simulink model "ship_template"  (R2021b)
settings: Solver=ode23t  StartTime=0.0  StopTime=60*2  MaxStep=0.1  RelTol=1e-3  AbsTol=1e-3
model workspace (MAT data in the model file):
  L = 1.2
  W = 1.2
undefined symbols (not defined in the file or in its folder): blue, blue0, blue1, blue2, centre, green, green0, green1, green2, left, Left, llx, lly, Mid, red, red0, red1, red2, right, Right, ulx, uly, X, Y, Z
libraries: sm_lib x278, nesl_utility x68, fl_lib x58, simulink x12, ee_lib x3, sdl_lib x3
(part 6 of 8)

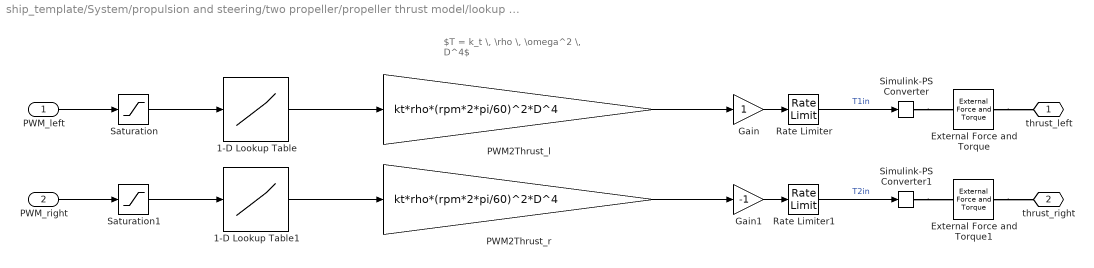
== system ship_template/System/propulsion and steering/two propeller/propeller thrust model/lookup model ==
  note: $T = k_t \, \rho \, \omega^2 \, D^4$
  PWM_left : Inport
  PWM_right : Inport  Port=2
  1-D Lookup Table : Lookup_n-D  NumberOfTableDimensions=1  BreakpointsForDimension1=[-1:0.1:1]  Table=tanh(3*[-1:0.1:1])  InternalRulePriority=Speed  RndMeth=Simplest  InputSameDT=on
  1-D Lookup Table1 : Lookup_n-D  NumberOfTableDimensions=1  BreakpointsForDimension1=[-1:0.1:1]  Table=tanh(3*[-1:0.1:1])  InternalRulePriority=Speed  RndMeth=Simplest  InputSameDT=on
  External Force and Torque : sm_lib/Forces and Torques/External Force and Torque  ForceResolutionFrame=AttachedFrame  EnableForceX=off  EnableForceY=off  EnableForceZ=on  EnableForce=off  TorqueResolutionFrame=AttachedFrame  EnableTorqueX=off  EnableTorqueY=off  EnableTorqueZ=off  EnableTorque=off
  External Force and Torque1 : sm_lib/Forces and Torques/External Force and Torque  ForceResolutionFrame=AttachedFrame  EnableForceX=off  EnableForceY=off  EnableForceZ=on  EnableForce=off  TorqueResolutionFrame=AttachedFrame  EnableTorqueX=off  EnableTorqueY=off  EnableTorqueZ=off  EnableTorque=off
  Gain : Gain
  Gain1 : Gain  Gain=-1
  PWM2Thrust_l : Gain  Gain=kt*rho*(rpm*2*pi/60)^2*D^4
  PWM2Thrust_r : Gain  Gain=kt*rho*(rpm*2*pi/60)^2*D^4
  Rate Limiter : RateLimiter  SampleTimeMode=inherited
  Rate Limiter1 : RateLimiter  SampleTimeMode=inherited
  Saturation : Saturate  UpperLimit=1  LowerLimit=-1
  Saturation1 : Saturate  UpperLimit=1  LowerLimit=-1
  Simulink-PS Converter : nesl_utility/Simulink-PS Converter  PhysicalDomain=network_engine_domain  SubClassName=ps_input  LeftPortType=input  RightPortType=output  PseudoPeriodic=off  Frequencies=[]  NoiseDistribution=none  NoiseParameters=[]  Unit=1  AffineConversion=off  FilteringAndDerivatives=provide  SimscapeFilterOrder=1  InputFilterTimeConstant=0.001  UdotUserProvided=0
      settings: SourceProductBaseCode=PW,SS
  Simulink-PS Converter1 : nesl_utility/Simulink-PS Converter  PhysicalDomain=network_engine_domain  SubClassName=ps_input  LeftPortType=input  RightPortType=output  PseudoPeriodic=off  Frequencies=[]  NoiseDistribution=none  NoiseParameters=[]  Unit=1  AffineConversion=off  FilteringAndDerivatives=provide  SimscapeFilterOrder=1  InputFilterTimeConstant=0.001  UdotUserProvided=0
      settings: SourceProductBaseCode=PW,SS
  thrust_left : PMIOPort  Side=Right
  thrust_right : PMIOPort  Port=2  Side=Right
  wires:
  Rate Limiter1/1 -> Simulink-PS Converter1/1  "T2in"
  Rate Limiter/1 -> Simulink-PS Converter/1  "T1in"
  PWM2Thrust_l/1 -> Gain/1
  PWM2Thrust_r/1 -> Gain1/1
  Saturation1/1 -> 1-D Lookup Table1/1
  Saturation/1 -> 1-D Lookup Table/1
  Gain1/1 -> Rate Limiter1/1
  Gain/1 -> Rate Limiter/1
  PWM_right/1 -> Saturation1/1
  PWM_left/1 -> Saturation/1
  1-D Lookup Table/1 -> PWM2Thrust_l/1
  1-D Lookup Table1/1 -> PWM2Thrust_r/1
  connections:
  Simulink-PS Converter1/RConn1 -- External Force and Torque1/LConn1
  Simulink-PS Converter/RConn1 -- External Force and Torque/LConn1
  External Force and Torque1/RConn1 -- thrust_right/RConn1
  External Force and Torque/RConn1 -- thrust_left/RConn1

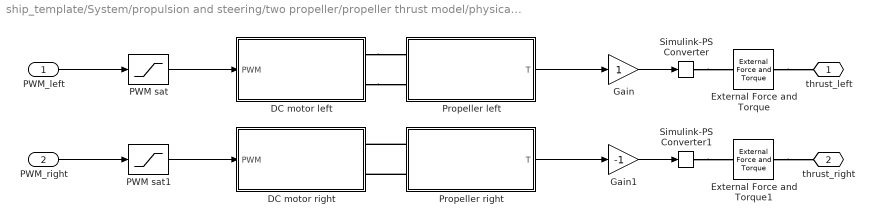
== system ship_template/System/propulsion and steering/two propeller/propeller thrust model/physical model ==
  PWM_left : Inport
  PWM_right : Inport  Port=2
  DC motor left : Subsystem
  DC motor right : Subsystem
  External Force and Torque : sm_lib/Forces and Torques/External Force and Torque  ForceResolutionFrame=AttachedFrame  EnableForceX=off  EnableForceY=off  EnableForceZ=on  EnableForce=off  TorqueResolutionFrame=AttachedFrame  EnableTorqueX=off  EnableTorqueY=off  EnableTorqueZ=off  EnableTorque=off
  External Force and Torque1 : sm_lib/Forces and Torques/External Force and Torque  ForceResolutionFrame=AttachedFrame  EnableForceX=off  EnableForceY=off  EnableForceZ=on  EnableForce=off  TorqueResolutionFrame=AttachedFrame  EnableTorqueX=off  EnableTorqueY=off  EnableTorqueZ=off  EnableTorque=off
  Gain : Gain
  Gain1 : Gain  Gain=-1
  PWM sat : Saturate  UpperLimit=1  LowerLimit=-1
  PWM sat1 : Saturate  UpperLimit=1  LowerLimit=-1
  Propeller left : Subsystem
  Propeller right : Subsystem
  Simulink-PS Converter : nesl_utility/Simulink-PS Converter  PhysicalDomain=network_engine_domain  SubClassName=ps_input  LeftPortType=input  RightPortType=output  PseudoPeriodic=off  Frequencies=[]  NoiseDistribution=none  NoiseParameters=[]  Unit=1  AffineConversion=off  FilteringAndDerivatives=provide  SimscapeFilterOrder=1  InputFilterTimeConstant=0.001  UdotUserProvided=0
      settings: SourceProductBaseCode=PW,SS
  Simulink-PS Converter1 : nesl_utility/Simulink-PS Converter  PhysicalDomain=network_engine_domain  SubClassName=ps_input  LeftPortType=input  RightPortType=output  PseudoPeriodic=off  Frequencies=[]  NoiseDistribution=none  NoiseParameters=[]  Unit=1  AffineConversion=off  FilteringAndDerivatives=provide  SimscapeFilterOrder=1  InputFilterTimeConstant=0.001  UdotUserProvided=0
      settings: SourceProductBaseCode=PW,SS
  thrust_left : PMIOPort  Side=Right
  thrust_right : PMIOPort  Port=2  Side=Right
  wires:
  Gain1/1 -> Simulink-PS Converter1/1
  Gain/1 -> Simulink-PS Converter/1
  PWM_left/1 -> PWM sat/1
  PWM sat/1 -> DC motor left/1(PWM)
  Propeller left/1(T) -> Gain/1
  PWM_right/1 -> PWM sat1/1
  PWM sat1/1 -> DC motor right/1(PWM)
  Propeller right/1(T) -> Gain1/1
  connections:
  Simulink-PS Converter1/RConn1 -- External Force and Torque1/LConn1
  Simulink-PS Converter/RConn1 -- External Force and Torque/LConn1
  External Force and Torque1/RConn1 -- thrust_right/RConn1
  External Force and Torque/RConn1 -- thrust_left/RConn1
  DC motor left/RConn1 -- Propeller left/LConn1
  DC motor left/RConn2 -- Propeller left/LConn2
  Propeller right/LConn2 -- DC motor right/RConn2
  Propeller right/LConn1 -- DC motor right/RConn1

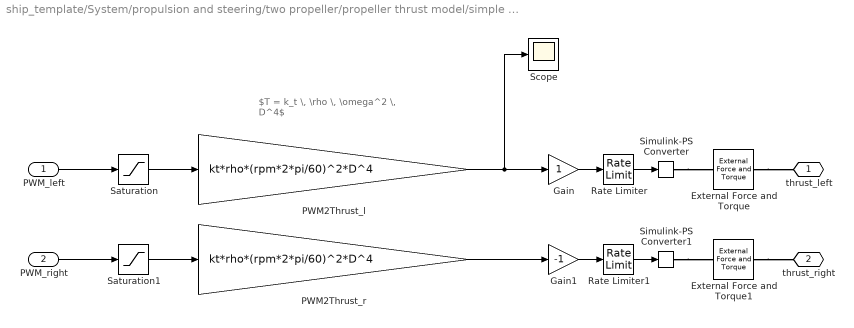
== system ship_template/System/propulsion and steering/two propeller/propeller thrust model/simple thrust ==
  note: $T = k_t \, \rho \, \omega^2 \, D^4$
  PWM_left : Inport
  PWM_right : Inport  Port=2
  External Force and Torque : sm_lib/Forces and Torques/External Force and Torque  ForceResolutionFrame=AttachedFrame  EnableForceX=off  EnableForceY=off  EnableForceZ=on  EnableForce=off  TorqueResolutionFrame=AttachedFrame  EnableTorqueX=off  EnableTorqueY=off  EnableTorqueZ=off  EnableTorque=off
  External Force and Torque1 : sm_lib/Forces and Torques/External Force and Torque  ForceResolutionFrame=AttachedFrame  EnableForceX=off  EnableForceY=off  EnableForceZ=on  EnableForce=off  TorqueResolutionFrame=AttachedFrame  EnableTorqueX=off  EnableTorqueY=off  EnableTorqueZ=off  EnableTorque=off
  Gain : Gain
  Gain1 : Gain  Gain=-1
  PWM2Thrust_l : Gain  Gain=kt*rho*(rpm*2*pi/60)^2*D^4
  PWM2Thrust_r : Gain  Gain=kt*rho*(rpm*2*pi/60)^2*D^4
  Rate Limiter : RateLimiter  SampleTimeMode=inherited
  Rate Limiter1 : RateLimiter  SampleTimeMode=inherited
  Saturation : Saturate  UpperLimit=1  LowerLimit=-1
  Saturation1 : Saturate  UpperLimit=1  LowerLimit=-1
  Scope : Scope
  Simulink-PS Converter : nesl_utility/Simulink-PS Converter  PhysicalDomain=network_engine_domain  SubClassName=ps_input  LeftPortType=input  RightPortType=output  PseudoPeriodic=off  Frequencies=[]  NoiseDistribution=none  NoiseParameters=[]  Unit=1  AffineConversion=off  FilteringAndDerivatives=provide  SimscapeFilterOrder=1  InputFilterTimeConstant=0.001  UdotUserProvided=0
      settings: SourceProductBaseCode=PW,SS
  Simulink-PS Converter1 : nesl_utility/Simulink-PS Converter  PhysicalDomain=network_engine_domain  SubClassName=ps_input  LeftPortType=input  RightPortType=output  PseudoPeriodic=off  Frequencies=[]  NoiseDistribution=none  NoiseParameters=[]  Unit=1  AffineConversion=off  FilteringAndDerivatives=provide  SimscapeFilterOrder=1  InputFilterTimeConstant=0.001  UdotUserProvided=0
      settings: SourceProductBaseCode=PW,SS
  thrust_left : PMIOPort  Side=Right
  thrust_right : PMIOPort  Port=2  Side=Right
  wires:
  PWM_left/1 -> Saturation/1
  PWM_right/1 -> Saturation1/1
  Gain/1 -> Rate Limiter/1
  Gain1/1 -> Rate Limiter1/1
  Saturation/1 -> PWM2Thrust_l/1
  Saturation1/1 -> PWM2Thrust_r/1
  PWM2Thrust_r/1 -> Gain1/1
  PWM2Thrust_l/1 -> Gain/1, Scope/1
  Rate Limiter/1 -> Simulink-PS Converter/1
  Rate Limiter1/1 -> Simulink-PS Converter1/1
  connections:
  External Force and Torque/RConn1 -- thrust_left/RConn1
  External Force and Torque1/RConn1 -- thrust_right/RConn1
  Simulink-PS Converter/RConn1 -- External Force and Torque/LConn1
  Simulink-PS Converter1/RConn1 -- External Force and Torque1/LConn1

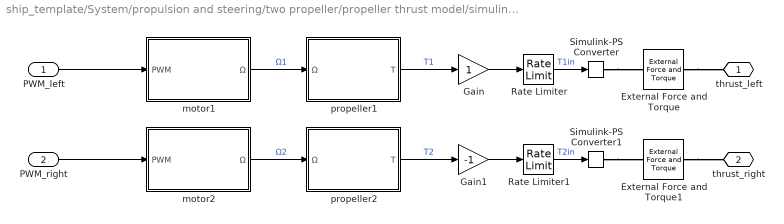
== system ship_template/System/propulsion and steering/two propeller/propeller thrust model/simulink model ==
  PWM_left : Inport
  PWM_right : Inport  Port=2
  External Force and Torque : sm_lib/Forces and Torques/External Force and Torque  ForceResolutionFrame=AttachedFrame  EnableForceX=off  EnableForceY=off  EnableForceZ=on  EnableForce=off  TorqueResolutionFrame=AttachedFrame  EnableTorqueX=off  EnableTorqueY=off  EnableTorqueZ=off  EnableTorque=off
  External Force and Torque1 : sm_lib/Forces and Torques/External Force and Torque  ForceResolutionFrame=AttachedFrame  EnableForceX=off  EnableForceY=off  EnableForceZ=on  EnableForce=off  TorqueResolutionFrame=AttachedFrame  EnableTorqueX=off  EnableTorqueY=off  EnableTorqueZ=off  EnableTorque=off
  Gain : Gain
  Gain1 : Gain  Gain=-1
  Rate Limiter : RateLimiter  SampleTimeMode=inherited
  Rate Limiter1 : RateLimiter  SampleTimeMode=inherited
  Simulink-PS Converter : nesl_utility/Simulink-PS Converter  PhysicalDomain=network_engine_domain  SubClassName=ps_input  LeftPortType=input  RightPortType=output  PseudoPeriodic=off  Frequencies=[]  NoiseDistribution=none  NoiseParameters=[]  Unit=1  AffineConversion=off  FilteringAndDerivatives=provide  SimscapeFilterOrder=1  InputFilterTimeConstant=0.001  UdotUserProvided=0
      settings: SourceProductBaseCode=PW,SS
  Simulink-PS Converter1 : nesl_utility/Simulink-PS Converter  PhysicalDomain=network_engine_domain  SubClassName=ps_input  LeftPortType=input  RightPortType=output  PseudoPeriodic=off  Frequencies=[]  NoiseDistribution=none  NoiseParameters=[]  Unit=1  AffineConversion=off  FilteringAndDerivatives=provide  SimscapeFilterOrder=1  InputFilterTimeConstant=0.001  UdotUserProvided=0
      settings: SourceProductBaseCode=PW,SS
  motor1 : Subsystem  mask(DC Motor){J=mprop*(D/2)^2, km=0.2, R=0.5, Vmax=7.2}
      mask prompts: J "Inertia, J [kgm^2]"; km "Motor constant, km [V*s/rad]"; R "Resistance, R [Ohm]"; Vmax "Maximum Voltage, Vmax [V]"
      mask help:
      | Circuit Dynamics:   PWM*Vmax == I*R + km*Ω
      | Rotor Dynamics:     J*dΩ/dt == km*I
      mask Display: image('$imagefile'); % Use "Edit Image" on toolstrip to change.
  motor2 : Subsystem  mask(DC Motor){J=mprop*(D/2)^2, km=0.2, R=0.5, Vmax=7.2}
      mask prompts: J "Inertia, J [kgm^2]"; km "Motor constant, km [V*s/rad]"; R "Resistance, R [Ohm]"; Vmax "Maximum Voltage, Vmax [V]"
      mask help:
      | Circuit Dynamics:   PWM*Vmax == I*R + km*Ω
      | Rotor Dynamics:     J*dΩ/dt == km*I
      mask Display: image('$imagefile'); % Use "Edit Image" on toolstrip to change.
  propeller1 : Subsystem  mask(Propeller Model){D=D, kt=kt, rho=rho}
      mask prompts: D "Propeller Diameter [m]"; kt "Thrust Coefficient"; rho "Fluid density [kg/m^3]"
      mask help: Propeller Dynamics: T = kt*rho*omega^2*D^4
      mask Display: image('$imagefile'); % Use "Edit Image" on toolstrip to change.
  propeller2 : Subsystem  mask(Propeller Model){D=D, kt=kt, rho=rho}
      mask prompts: D "Propeller Diameter [m]"; kt "Thrust Coefficient"; rho "Fluid density [kg/m^3]"
      mask help: Propeller Dynamics: T = kt*rho*omega^2*D^4
      mask Display: image('$imagefile'); % Use "Edit Image" on toolstrip to change.
  thrust_left : PMIOPort  Side=Right
  thrust_right : PMIOPort  Port=2  Side=Right
  wires:
  PWM_left/1 -> motor1/1(PWM)
  PWM_right/1 -> motor2/1(PWM)
  Rate Limiter/1 -> Simulink-PS Converter/1  "T1in"
  Rate Limiter1/1 -> Simulink-PS Converter1/1  "T2in"
  motor1/1(Ω) -> propeller1/1(Ω)  "Ω1"
  motor2/1(Ω) -> propeller2/1(Ω)  "Ω2"
  propeller2/1(T) -> Gain1/1  "T2"
  propeller1/1(T) -> Gain/1  "T1"
  Gain/1 -> Rate Limiter/1
  Gain1/1 -> Rate Limiter1/1
  connections:
  External Force and Torque/RConn1 -- thrust_left/RConn1
  External Force and Torque1/RConn1 -- thrust_right/RConn1
  Simulink-PS Converter/RConn1 -- External Force and Torque/LConn1
  Simulink-PS Converter1/RConn1 -- External Force and Torque1/LConn1

== system ship_template/System/ship to world joint/nonlinear_drag/Drag model/rotational_drag_model_theta ==
  PS Abs : fl_lib/Physical Signals/Nonlinear Operators/PS Abs
      settings: SourceProductBaseCode=SS  InternalSimscapePortConfiguration="{\"Bottom\":[],\"Left\":[{\"id\":\"I\",\"label\":\"\",\"type\":\"input\"}],\"Right\":[{\"id\":\"O\",\"label\":\"\",\"type\":\"output\"}],\"Top\":[]}"
  PS Gain : fl_lib/Physical Signals/Functions/PS Gain  gain=1/2*Cd*rho*A^4*R kg*m^2/rad^2
  PS Product : fl_lib/Physical Signals/Functions/PS Product
  f : PMIOPort  Side=Right
  v : PMIOPort  Port=2  Side=Left
  connections:
  PS Gain/LConn1 -- PS Product/RConn1
  PS Product/LConn2 -- PS Abs/RConn1
  PS Product/LConn1 -- PS Abs/LConn1 -- v/RConn1
  f/RConn1 -- PS Gain/RConn1

== system ship_template/System/ship to world joint/nonlinear_drag/Drag model/translational_drag_model_x ==
  PS Abs : fl_lib/Physical Signals/Nonlinear Operators/PS Abs
      settings: SourceProductBaseCode=SS  InternalSimscapePortConfiguration="{\"Bottom\":[],\"Left\":[{\"id\":\"I\",\"label\":\"\",\"type\":\"input\"}],\"Right\":[{\"id\":\"O\",\"label\":\"\",\"type\":\"output\"}],\"Top\":[]}"
  PS Gain : fl_lib/Physical Signals/Functions/PS Gain  gain=1/2*Cd*rho*A kg/m
  PS Product : fl_lib/Physical Signals/Functions/PS Product
  f : PMIOPort  Side=Right
  v : PMIOPort  Port=2  Side=Left
  connections:
  PS Gain/LConn1 -- PS Product/RConn1
  PS Product/LConn2 -- PS Abs/RConn1
  PS Abs/LConn1 -- v/RConn1 -- PS Product/LConn1
  f/RConn1 -- PS Gain/RConn1

== system ship_template/System/ship to world joint/nonlinear_drag/Drag model/translational_drag_model_y ==
  PS Abs : fl_lib/Physical Signals/Nonlinear Operators/PS Abs
      settings: SourceProductBaseCode=SS  InternalSimscapePortConfiguration="{\"Bottom\":[],\"Left\":[{\"id\":\"I\",\"label\":\"\",\"type\":\"input\"}],\"Right\":[{\"id\":\"O\",\"label\":\"\",\"type\":\"output\"}],\"Top\":[]}"
  PS Gain : fl_lib/Physical Signals/Functions/PS Gain  gain=1/2*Cd*rho*A kg/m
  PS Product : fl_lib/Physical Signals/Functions/PS Product
  f : PMIOPort  Side=Right
  v : PMIOPort  Port=2  Side=Left
  connections:
  f/RConn1 -- PS Gain/RConn1
  v/RConn1 -- PS Abs/LConn1 -- PS Product/LConn1
  PS Product/LConn2 -- PS Abs/RConn1
  PS Gain/LConn1 -- PS Product/RConn1

== system ship_template/System/object scenario/3objs/contact models/tank2collector/Subsystem ==
  Simscape Bus11 : SimscapeBus  HierarchyStrings=llx;ulx;lly;uly
  Spatial Contact Force{1,12,16..17} (4 alike) : sm_lib/Forces and Torques/Spatial Contact Force  CoefficientOfDynamicFriction=0.3  CoefficientOfStaticFriction=0.5  SenseContactBaseRotation=off  SenseContactBaseTranslation=off  NormalDamping=b  NormalDampingUnits=N/(m/s)  SenseContactFollowerRotation=off  SenseContactFollowerTranslation=off  SenseContactSignal=off  NormalStiffness=k  NormalStiffnessUnits=N/m  FrictionalCriticalVelocity=1e-3  FrictionalCriticalVelocityUnits=m/s  ZeroCrossDetectContactStartAndEnd=off  FrictionType=SmoothStickSlip  SenseFrictionalForceMagnitude=off  SenseNormalForceMagnitude=off  NormalForceType=SmoothSpringDamper  SenseNormalVelocity=off  SenseSeparationDistance=off  SenseTangentialVelocity=off  SenseTangentialVelocityMagnitude=off  NormalTransitionRegionWidth=x  NormalTransitionRegionWidthUnits=m
  tank wall : PMIOPort  Side=Left
  F : PMIOPort  Port=2  Side=Right
  connections:
  Simscape Bus11/LConn3 -- Spatial Contact Force16/LConn1
  Spatial Contact Force17/LConn1 -- Simscape Bus11/LConn1
  Spatial Contact Force16/RConn1 -- Spatial Contact Force1/RConn1 -- F/RConn1 -- Spatial Contact Force17/RConn1 -- Spatial Contact Force12/RConn1
  Simscape Bus11/LConn4 -- Spatial Contact Force1/LConn1
  tank wall/RConn1 -- Simscape Bus11/RConn1
  Simscape Bus11/LConn2 -- Spatial Contact Force12/LConn1

== system ship_template/System/object scenario/3objs/contact models/tank2collector/Subsystem1 ==
  Simscape Bus11 : SimscapeBus  HierarchyStrings=llx;ulx;lly;uly
  Spatial Contact Force{1,12,16..17} (4 alike) : sm_lib/Forces and Torques/Spatial Contact Force  CoefficientOfDynamicFriction=0.3  CoefficientOfStaticFriction=0.5  SenseContactBaseRotation=off  SenseContactBaseTranslation=off  NormalDamping=b  NormalDampingUnits=N/(m/s)  SenseContactFollowerRotation=off  SenseContactFollowerTranslation=off  SenseContactSignal=off  NormalStiffness=k  NormalStiffnessUnits=N/m  FrictionalCriticalVelocity=1e-3  FrictionalCriticalVelocityUnits=m/s  ZeroCrossDetectContactStartAndEnd=off  FrictionType=SmoothStickSlip  SenseFrictionalForceMagnitude=off  SenseNormalForceMagnitude=off  NormalForceType=SmoothSpringDamper  SenseNormalVelocity=off  SenseSeparationDistance=off  SenseTangentialVelocity=off  SenseTangentialVelocityMagnitude=off  NormalTransitionRegionWidth=x  NormalTransitionRegionWidthUnits=m
  tank wall : PMIOPort  Side=Left
  F : PMIOPort  Port=2  Side=Right
  connections:
  Simscape Bus11/LConn2 -- Spatial Contact Force12/LConn1
  tank wall/RConn1 -- Simscape Bus11/RConn1
  Simscape Bus11/LConn4 -- Spatial Contact Force1/LConn1
  F/RConn1 -- Spatial Contact Force12/RConn1 -- Spatial Contact Force17/RConn1 -- Spatial Contact Force16/RConn1 -- Spatial Contact Force1/RConn1
  Spatial Contact Force17/LConn1 -- Simscape Bus11/LConn1
  Simscape Bus11/LConn3 -- Spatial Contact Force16/LConn1

== system ship_template/System/object scenario/3objs/contact models/tank2collector/Subsystem2 ==
  Simscape Bus11 : SimscapeBus  HierarchyStrings=llx;ulx;lly;uly
  Spatial Contact Force{1,12,16..17} (4 alike) : sm_lib/Forces and Torques/Spatial Contact Force  CoefficientOfDynamicFriction=0.3  CoefficientOfStaticFriction=0.5  SenseContactBaseRotation=off  SenseContactBaseTranslation=off  NormalDamping=b  NormalDampingUnits=N/(m/s)  SenseContactFollowerRotation=off  SenseContactFollowerTranslation=off  SenseContactSignal=off  NormalStiffness=k  NormalStiffnessUnits=N/m  FrictionalCriticalVelocity=1e-3  FrictionalCriticalVelocityUnits=m/s  ZeroCrossDetectContactStartAndEnd=off  FrictionType=SmoothStickSlip  SenseFrictionalForceMagnitude=off  SenseNormalForceMagnitude=off  NormalForceType=SmoothSpringDamper  SenseNormalVelocity=off  SenseSeparationDistance=off  SenseTangentialVelocity=off  SenseTangentialVelocityMagnitude=off  NormalTransitionRegionWidth=x  NormalTransitionRegionWidthUnits=m
  tank wall : PMIOPort  Side=Left
  F : PMIOPort  Port=2  Side=Right
  connections:
  Simscape Bus11/LConn3 -- Spatial Contact Force16/LConn1
  Spatial Contact Force17/LConn1 -- Simscape Bus11/LConn1
  Spatial Contact Force1/RConn1 -- Spatial Contact Force16/RConn1 -- Spatial Contact Force17/RConn1 -- Spatial Contact Force12/RConn1 -- F/RConn1
  Simscape Bus11/LConn4 -- Spatial Contact Force1/LConn1
  tank wall/RConn1 -- Simscape Bus11/RConn1
  Simscape Bus11/LConn2 -- Spatial Contact Force12/LConn1

== system ship_template/System/object scenario/3objs/objects/object location/checkCollected ==
  xy : Inport
  Compare To Constant : simulink/Logic and Bit Operations/Compare To Constant  relop=<=  const=homeRadius  OutDataTypeStr=boolean
  Constant : Constant  Value=[Xhome, Yhome]
  Sqrt : Sqrt  SaturateOnIntegerOverflow=on
  Square : Math  Operator=square  SaturateOnIntegerOverflow=on
  Sum : Sum  Inputs=|-+
  Sum of Elements : Sum  Inputs=+
  collectFlag : Outport
  wires:
  Sum of Elements/1 -> Sqrt/1
  Sqrt/1 -> Compare To Constant/1  "dist"
  xy/1 -> Sum/1
  Square/1 -> Sum of Elements/1
  Compare To Constant/1 -> collectFlag/1  "collected"
  Constant/1 -> Sum/2
  Sum/1 -> Square/1

== system ship_template/System/object scenario/3objs/objects/object location/checkCollected1 ==
  xy : Inport
  Compare To Constant : simulink/Logic and Bit Operations/Compare To Constant  relop=<=  const=homeRadius  OutDataTypeStr=boolean
  Constant : Constant  Value=[Xhome, Yhome]
  Sqrt : Sqrt  SaturateOnIntegerOverflow=on
  Square : Math  Operator=square  SaturateOnIntegerOverflow=on
  Sum : Sum  Inputs=|-+
  Sum of Elements : Sum  Inputs=+
  collectFlag : Outport
  wires:
  Sum/1 -> Square/1
  Constant/1 -> Sum/2
  Compare To Constant/1 -> collectFlag/1  "collected"
  Square/1 -> Sum of Elements/1
  xy/1 -> Sum/1
  Sqrt/1 -> Compare To Constant/1  "dist"
  Sum of Elements/1 -> Sqrt/1

== system ship_template/System/object scenario/3objs/objects/object location/checkCollected2 ==
  xy : Inport
  Compare To Constant : simulink/Logic and Bit Operations/Compare To Constant  relop=<=  const=homeRadius  OutDataTypeStr=boolean
  Constant : Constant  Value=[Xhome, Yhome]
  Sqrt : Sqrt  SaturateOnIntegerOverflow=on
  Square : Math  Operator=square  SaturateOnIntegerOverflow=on
  Sum : Sum  Inputs=|-+
  Sum of Elements : Sum  Inputs=+
  collectFlag : Outport
  wires:
  Sum of Elements/1 -> Sqrt/1
  Sqrt/1 -> Compare To Constant/1  "dist"
  xy/1 -> Sum/1
  Square/1 -> Sum of Elements/1
  Compare To Constant/1 -> collectFlag/1  "collected"
  Constant/1 -> Sum/2
  Sum/1 -> Square/1

== system ship_template/System/object scenario/3objs/objects/object location/transform sensor ==
  Mux1 : Mux  Inputs=2
  PS-Simulink Converter : nesl_utility/PS-Simulink Converter  PhysicalDomain=network_engine_domain  SubClassName=ps_output  LeftPortType=input  RightPortType=output  PseudoPeriodic=off  Frequencies=[]  Unit=inherit  AffineConversion=off
      settings: SourceProductBaseCode=PW,SS
  PS-Simulink Converter1 : nesl_utility/PS-Simulink Converter  PhysicalDomain=network_engine_domain  SubClassName=ps_output  LeftPortType=input  RightPortType=output  PseudoPeriodic=off  Frequencies=[]  Unit=inherit  AffineConversion=off
      settings: SourceProductBaseCode=PW,SS
  Transform Sensor : sm_lib/Frames and Transforms/Transform Sensor  MeasurementFrame=World  SenseAngle=off  SenseAxis=off  SenseAngle1=off  SenseAngle2=off  SenseAngle3=off  SenseQ=off  SenseR=off  SenseOmegaX=off  SenseOmegaY=off  SenseOmegaZ=off  SenseOmega1=off  SenseOmega2=off  SenseOmega3=off  SenseQDot=off  SenseRDot=off  SenseAlphaX=off  SenseAlphaY=off  SenseAlphaZ=off  SenseAlpha1=off  SenseAlpha2=off  SenseAlpha3=off  SenseQDDot=off  SenseRDDot=off  SenseX=on  SenseY=on  SenseZ=off  SenseRad=off  SenseAzim=off  SenseDist=off  SenseInc=off  SenseXDot=off  SenseYDot=off  SenseZDot=off  SenseRadDot=off  SenseAzimDot=off  SenseDistDot=off  SenseIncDot=off  SenseXDDot=off  SenseYDDot=off  SenseZDDot=off  SenseRadDDot=off  SenseAzimDDot=off  SenseDistDDot=off  SenseIncDDot=off
  WF : PMIOPort  Side=Left
  F : PMIOPort  Port=2  Side=Right
  xy : Outport
  wires:
  PS-Simulink Converter1/1 -> Mux1/2
  Mux1/1 -> xy/1
  PS-Simulink Converter/1 -> Mux1/1
  connections:
  PS-Simulink Converter1/LConn1 -- Transform Sensor/RConn3
  PS-Simulink Converter/LConn1 -- Transform Sensor/RConn2
  WF/RConn1 -- Transform Sensor/LConn1
  Transform Sensor/RConn1 -- F/RConn1

== system ship_template/System/object scenario/3objs/objects/object location/transform sensor1 ==
  Mux1 : Mux  Inputs=2
  PS-Simulink Converter : nesl_utility/PS-Simulink Converter  PhysicalDomain=network_engine_domain  SubClassName=ps_output  LeftPortType=input  RightPortType=output  PseudoPeriodic=off  Frequencies=[]  Unit=inherit  AffineConversion=off
      settings: SourceProductBaseCode=PW,SS
  PS-Simulink Converter1 : nesl_utility/PS-Simulink Converter  PhysicalDomain=network_engine_domain  SubClassName=ps_output  LeftPortType=input  RightPortType=output  PseudoPeriodic=off  Frequencies=[]  Unit=inherit  AffineConversion=off
      settings: SourceProductBaseCode=PW,SS
  Transform Sensor : sm_lib/Frames and Transforms/Transform Sensor  MeasurementFrame=World  SenseAngle=off  SenseAxis=off  SenseAngle1=off  SenseAngle2=off  SenseAngle3=off  SenseQ=off  SenseR=off  SenseOmegaX=off  SenseOmegaY=off  SenseOmegaZ=off  SenseOmega1=off  SenseOmega2=off  SenseOmega3=off  SenseQDot=off  SenseRDot=off  SenseAlphaX=off  SenseAlphaY=off  SenseAlphaZ=off  SenseAlpha1=off  SenseAlpha2=off  SenseAlpha3=off  SenseQDDot=off  SenseRDDot=off  SenseX=on  SenseY=on  SenseZ=off  SenseRad=off  SenseAzim=off  SenseDist=off  SenseInc=off  SenseXDot=off  SenseYDot=off  SenseZDot=off  SenseRadDot=off  SenseAzimDot=off  SenseDistDot=off  SenseIncDot=off  SenseXDDot=off  SenseYDDot=off  SenseZDDot=off  SenseRadDDot=off  SenseAzimDDot=off  SenseDistDDot=off  SenseIncDDot=off
  WF : PMIOPort  Side=Left
  F : PMIOPort  Port=2  Side=Right
  xy : Outport
  wires:
  PS-Simulink Converter/1 -> Mux1/1
  Mux1/1 -> xy/1
  PS-Simulink Converter1/1 -> Mux1/2
  connections:
  Transform Sensor/RConn1 -- F/RConn1
  WF/RConn1 -- Transform Sensor/LConn1
  PS-Simulink Converter/LConn1 -- Transform Sensor/RConn2
  PS-Simulink Converter1/LConn1 -- Transform Sensor/RConn3

== system ship_template/System/object scenario/3objs/objects/object location/transform sensor2 ==
  Mux1 : Mux  Inputs=2
  PS-Simulink Converter : nesl_utility/PS-Simulink Converter  PhysicalDomain=network_engine_domain  SubClassName=ps_output  LeftPortType=input  RightPortType=output  PseudoPeriodic=off  Frequencies=[]  Unit=inherit  AffineConversion=off
      settings: SourceProductBaseCode=PW,SS
  PS-Simulink Converter1 : nesl_utility/PS-Simulink Converter  PhysicalDomain=network_engine_domain  SubClassName=ps_output  LeftPortType=input  RightPortType=output  PseudoPeriodic=off  Frequencies=[]  Unit=inherit  AffineConversion=off
      settings: SourceProductBaseCode=PW,SS
  Transform Sensor : sm_lib/Frames and Transforms/Transform Sensor  MeasurementFrame=World  SenseAngle=off  SenseAxis=off  SenseAngle1=off  SenseAngle2=off  SenseAngle3=off  SenseQ=off  SenseR=off  SenseOmegaX=off  SenseOmegaY=off  SenseOmegaZ=off  SenseOmega1=off  SenseOmega2=off  SenseOmega3=off  SenseQDot=off  SenseRDot=off  SenseAlphaX=off  SenseAlphaY=off  SenseAlphaZ=off  SenseAlpha1=off  SenseAlpha2=off  SenseAlpha3=off  SenseQDDot=off  SenseRDDot=off  SenseX=on  SenseY=on  SenseZ=off  SenseRad=off  SenseAzim=off  SenseDist=off  SenseInc=off  SenseXDot=off  SenseYDot=off  SenseZDot=off  SenseRadDot=off  SenseAzimDot=off  SenseDistDot=off  SenseIncDot=off  SenseXDDot=off  SenseYDDot=off  SenseZDDot=off  SenseRadDDot=off  SenseAzimDDot=off  SenseDistDDot=off  SenseIncDDot=off
  WF : PMIOPort  Side=Left
  F : PMIOPort  Port=2  Side=Right
  xy : Outport
  wires:
  PS-Simulink Converter1/1 -> Mux1/2
  Mux1/1 -> xy/1
  PS-Simulink Converter/1 -> Mux1/1
  connections:
  PS-Simulink Converter1/LConn1 -- Transform Sensor/RConn3
  PS-Simulink Converter/LConn1 -- Transform Sensor/RConn2
  WF/RConn1 -- Transform Sensor/LConn1
  Transform Sensor/RConn1 -- F/RConn1

== system ship_template/System/object scenario/9objs/contact models/object2collector/objectcontact ==
  Simscape Bus1 : SimscapeBus  HierarchyStrings=blue0;green0;red0;blue1;green1;red1;blue2;green2;red2
  Spatial Contact Force{1..6,9..11} (9 alike) : sm_lib/Forces and Torques/Spatial Contact Force  CoefficientOfDynamicFriction=0.3  CoefficientOfStaticFriction=0.5  SenseContactBaseRotation=off  SenseContactBaseTranslation=off  NormalDamping=b  NormalDampingUnits=N/(m/s)  SenseContactFollowerRotation=off  SenseContactFollowerTranslation=off  SenseContactSignal=off  NormalStiffness=k  NormalStiffnessUnits=N/m  FrictionalCriticalVelocity=1e-3  FrictionalCriticalVelocityUnits=m/s  ZeroCrossDetectContactStartAndEnd=off  FrictionType=SmoothStickSlip  SenseFrictionalForceMagnitude=off  SenseNormalForceMagnitude=off  NormalForceType=SmoothSpringDamper  SenseNormalVelocity=off  SenseSeparationDistance=off  SenseTangentialVelocity=off  SenseTangentialVelocityMagnitude=off  NormalTransitionRegionWidth=x  NormalTransitionRegionWidthUnits=m
  object : PMIOPort  Side=Left
  F : PMIOPort  Port=2  Side=Right
  connections:
  Spatial Contact Force9/RConn1 -- Spatial Contact Force2/RConn1 -- Spatial Contact Force3/RConn1 -- Spatial Contact Force1/RConn1 -- Spatial Contact Force5/RConn1 -- Spatial Contact Force4/RConn1 -- Spatial Contact Force6/RConn1 -- Spatial Contact Force11/RConn1 -- Spatial Contact Force10/RConn1 -- F/RConn1
  Spatial Contact Force10/LConn1 -- Simscape Bus1/LConn5
  Spatial Contact Force2/LConn1 -- Simscape Bus1/LConn3
  Spatial Contact Force3/LConn1 -- Simscape Bus1/LConn1
  Spatial Contact Force11/LConn1 -- Simscape Bus1/LConn6
  Spatial Contact Force1/LConn1 -- Simscape Bus1/LConn2
  Spatial Contact Force4/LConn1 -- Simscape Bus1/LConn8
  Spatial Contact Force9/LConn1 -- Simscape Bus1/LConn4
  Spatial Contact Force5/LConn1 -- Simscape Bus1/LConn9
  Spatial Contact Force6/LConn1 -- Simscape Bus1/LConn7
  Simscape Bus1/RConn1 -- object/RConn1

== system ship_template/System/object scenario/9objs/contact models/object2collector/objectcontact1 ==
  Simscape Bus1 : SimscapeBus  HierarchyStrings=blue0;green0;red0;blue1;green1;red1;blue2;green2;red2
  Spatial Contact Force{1..6,9..11} (9 alike) : sm_lib/Forces and Torques/Spatial Contact Force  CoefficientOfDynamicFriction=0.3  CoefficientOfStaticFriction=0.5  SenseContactBaseRotation=off  SenseContactBaseTranslation=off  NormalDamping=b  NormalDampingUnits=N/(m/s)  SenseContactFollowerRotation=off  SenseContactFollowerTranslation=off  SenseContactSignal=off  NormalStiffness=k  NormalStiffnessUnits=N/m  FrictionalCriticalVelocity=1e-3  FrictionalCriticalVelocityUnits=m/s  ZeroCrossDetectContactStartAndEnd=off  FrictionType=SmoothStickSlip  SenseFrictionalForceMagnitude=off  SenseNormalForceMagnitude=off  NormalForceType=SmoothSpringDamper  SenseNormalVelocity=off  SenseSeparationDistance=off  SenseTangentialVelocity=off  SenseTangentialVelocityMagnitude=off  NormalTransitionRegionWidth=x  NormalTransitionRegionWidthUnits=m
  object : PMIOPort  Side=Left
  F : PMIOPort  Port=2  Side=Right
  connections:
  Simscape Bus1/RConn1 -- object/RConn1
  Spatial Contact Force6/LConn1 -- Simscape Bus1/LConn7
  Spatial Contact Force5/LConn1 -- Simscape Bus1/LConn9
  Spatial Contact Force9/LConn1 -- Simscape Bus1/LConn4
  Spatial Contact Force4/LConn1 -- Simscape Bus1/LConn8
  Spatial Contact Force1/LConn1 -- Simscape Bus1/LConn2
  Spatial Contact Force11/LConn1 -- Simscape Bus1/LConn6
  Spatial Contact Force3/LConn1 -- Simscape Bus1/LConn1
  Spatial Contact Force2/LConn1 -- Simscape Bus1/LConn3
  Spatial Contact Force10/LConn1 -- Simscape Bus1/LConn5
  F/RConn1 -- Spatial Contact Force10/RConn1 -- Spatial Contact Force11/RConn1 -- Spatial Contact Force6/RConn1 -- Spatial Contact Force4/RConn1 -- Spatial Contact Force5/RConn1 -- Spatial Contact Force1/RConn1 -- Spatial Contact Force3/RConn1 -- Spatial Contact Force2/RConn1 -- Spatial Contact Force9/RConn1

== system ship_template/System/object scenario/9objs/contact models/object2collector/objectcontact2 ==
  Simscape Bus1 : SimscapeBus  HierarchyStrings=blue0;green0;red0;blue1;green1;red1;blue2;green2;red2
  Spatial Contact Force{1..6,9..11} (9 alike) : sm_lib/Forces and Torques/Spatial Contact Force  CoefficientOfDynamicFriction=0.3  CoefficientOfStaticFriction=0.5  SenseContactBaseRotation=off  SenseContactBaseTranslation=off  NormalDamping=b  NormalDampingUnits=N/(m/s)  SenseContactFollowerRotation=off  SenseContactFollowerTranslation=off  SenseContactSignal=off  NormalStiffness=k  NormalStiffnessUnits=N/m  FrictionalCriticalVelocity=1e-3  FrictionalCriticalVelocityUnits=m/s  ZeroCrossDetectContactStartAndEnd=off  FrictionType=SmoothStickSlip  SenseFrictionalForceMagnitude=off  SenseNormalForceMagnitude=off  NormalForceType=SmoothSpringDamper  SenseNormalVelocity=off  SenseSeparationDistance=off  SenseTangentialVelocity=off  SenseTangentialVelocityMagnitude=off  NormalTransitionRegionWidth=x  NormalTransitionRegionWidthUnits=m
  object : PMIOPort  Side=Left
  F : PMIOPort  Port=2  Side=Right
  connections:
  Spatial Contact Force9/RConn1 -- Spatial Contact Force2/RConn1 -- Spatial Contact Force3/RConn1 -- Spatial Contact Force1/RConn1 -- Spatial Contact Force5/RConn1 -- Spatial Contact Force4/RConn1 -- Spatial Contact Force6/RConn1 -- Spatial Contact Force11/RConn1 -- Spatial Contact Force10/RConn1 -- F/RConn1
  Spatial Contact Force10/LConn1 -- Simscape Bus1/LConn5
  Spatial Contact Force2/LConn1 -- Simscape Bus1/LConn3
  Spatial Contact Force3/LConn1 -- Simscape Bus1/LConn1
  Spatial Contact Force11/LConn1 -- Simscape Bus1/LConn6
  Spatial Contact Force1/LConn1 -- Simscape Bus1/LConn2
  Spatial Contact Force4/LConn1 -- Simscape Bus1/LConn8
  Spatial Contact Force9/LConn1 -- Simscape Bus1/LConn4
  Spatial Contact Force5/LConn1 -- Simscape Bus1/LConn9
  Spatial Contact Force6/LConn1 -- Simscape Bus1/LConn7
  Simscape Bus1/RConn1 -- object/RConn1

== system ship_template/System/object scenario/9objs/contact models/object2object/objectcontact ==
  Simscape Bus1 : SimscapeBus  HierarchyStrings=green0;red0;blue1;green1;red1;blue2;green2;red2
  Spatial Contact Force{1..2,4..6,9..11} (8 alike) : sm_lib/Forces and Torques/Spatial Contact Force  CoefficientOfDynamicFriction=0.3  CoefficientOfStaticFriction=0.5  SenseContactBaseRotation=off  SenseContactBaseTranslation=off  NormalDamping=b  NormalDampingUnits=N/(m/s)  SenseContactFollowerRotation=off  SenseContactFollowerTranslation=off  SenseContactSignal=off  NormalStiffness=k  NormalStiffnessUnits=N/m  FrictionalCriticalVelocity=1e-3  FrictionalCriticalVelocityUnits=m/s  ZeroCrossDetectContactStartAndEnd=off  FrictionType=SmoothStickSlip  SenseFrictionalForceMagnitude=off  SenseNormalForceMagnitude=off  NormalForceType=SmoothSpringDamper  SenseNormalVelocity=off  SenseSeparationDistance=off  SenseTangentialVelocity=off  SenseTangentialVelocityMagnitude=off  NormalTransitionRegionWidth=x  NormalTransitionRegionWidthUnits=m
  object : PMIOPort  Side=Left
  F : PMIOPort  Port=2  Side=Right
  connections:
  Spatial Contact Force9/RConn1 -- Spatial Contact Force5/RConn1 -- Spatial Contact Force4/RConn1 -- Spatial Contact Force6/RConn1 -- Spatial Contact Force11/RConn1 -- F/RConn1 -- Spatial Contact Force10/RConn1 -- Spatial Contact Force2/RConn1 -- Spatial Contact Force1/RConn1
  Spatial Contact Force10/LConn1 -- Simscape Bus1/LConn4
  Spatial Contact Force2/LConn1 -- Simscape Bus1/LConn2
  Spatial Contact Force11/LConn1 -- Simscape Bus1/LConn5
  Spatial Contact Force1/LConn1 -- Simscape Bus1/LConn1
  Spatial Contact Force4/LConn1 -- Simscape Bus1/LConn7
  Spatial Contact Force9/LConn1 -- Simscape Bus1/LConn3
  Spatial Contact Force5/LConn1 -- Simscape Bus1/LConn8
  Spatial Contact Force6/LConn1 -- Simscape Bus1/LConn6
  Simscape Bus1/RConn1 -- object/RConn1

== system ship_template/System/object scenario/9objs/contact models/object2object/objectcontact1 ==
  Simscape Bus1 : SimscapeBus  HierarchyStrings=red0;blue1;green1;red1;blue2;green2;red2
  Spatial Contact Force{2,4..6,9..11} (7 alike) : sm_lib/Forces and Torques/Spatial Contact Force  CoefficientOfDynamicFriction=0.3  CoefficientOfStaticFriction=0.5  SenseContactBaseRotation=off  SenseContactBaseTranslation=off  NormalDamping=b  NormalDampingUnits=N/(m/s)  SenseContactFollowerRotation=off  SenseContactFollowerTranslation=off  SenseContactSignal=off  NormalStiffness=k  NormalStiffnessUnits=N/m  FrictionalCriticalVelocity=1e-3  FrictionalCriticalVelocityUnits=m/s  ZeroCrossDetectContactStartAndEnd=off  FrictionType=SmoothStickSlip  SenseFrictionalForceMagnitude=off  SenseNormalForceMagnitude=off  NormalForceType=SmoothSpringDamper  SenseNormalVelocity=off  SenseSeparationDistance=off  SenseTangentialVelocity=off  SenseTangentialVelocityMagnitude=off  NormalTransitionRegionWidth=x  NormalTransitionRegionWidthUnits=m
  object : PMIOPort  Side=Left
  F : PMIOPort  Port=2  Side=Right
  connections:
  Simscape Bus1/RConn1 -- object/RConn1
  Spatial Contact Force6/LConn1 -- Simscape Bus1/LConn5
  Spatial Contact Force5/LConn1 -- Simscape Bus1/LConn7
  Spatial Contact Force9/LConn1 -- Simscape Bus1/LConn2
  Spatial Contact Force4/LConn1 -- Simscape Bus1/LConn6
  Spatial Contact Force11/LConn1 -- Simscape Bus1/LConn4
  Spatial Contact Force2/LConn1 -- Simscape Bus1/LConn1
  Spatial Contact Force10/LConn1 -- Simscape Bus1/LConn3
  F/RConn1 -- Spatial Contact Force2/RConn1 -- Spatial Contact Force9/RConn1 -- Spatial Contact Force10/RConn1 -- Spatial Contact Force11/RConn1 -- Spatial Contact Force6/RConn1 -- Spatial Contact Force4/RConn1 -- Spatial Contact Force5/RConn1

== system ship_template/System/object scenario/9objs/contact models/object2object/objectcontact2 ==
  Simscape Bus1 : SimscapeBus  HierarchyStrings=blue1;green1;red1;blue2;green2;red2
  Spatial Contact Force{4..6,9..11} (6 alike) : sm_lib/Forces and Torques/Spatial Contact Force  CoefficientOfDynamicFriction=0.3  CoefficientOfStaticFriction=0.5  SenseContactBaseRotation=off  SenseContactBaseTranslation=off  NormalDamping=b  NormalDampingUnits=N/(m/s)  SenseContactFollowerRotation=off  SenseContactFollowerTranslation=off  SenseContactSignal=off  NormalStiffness=k  NormalStiffnessUnits=N/m  FrictionalCriticalVelocity=1e-3  FrictionalCriticalVelocityUnits=m/s  ZeroCrossDetectContactStartAndEnd=off  FrictionType=SmoothStickSlip  SenseFrictionalForceMagnitude=off  SenseNormalForceMagnitude=off  NormalForceType=SmoothSpringDamper  SenseNormalVelocity=off  SenseSeparationDistance=off  SenseTangentialVelocity=off  SenseTangentialVelocityMagnitude=off  NormalTransitionRegionWidth=x  NormalTransitionRegionWidthUnits=m
  object : PMIOPort  Side=Left
  F : PMIOPort  Port=2  Side=Right
  connections:
  Spatial Contact Force9/RConn1 -- Spatial Contact Force5/RConn1 -- Spatial Contact Force4/RConn1 -- Spatial Contact Force6/RConn1 -- F/RConn1 -- Spatial Contact Force11/RConn1 -- Spatial Contact Force10/RConn1
  Spatial Contact Force10/LConn1 -- Simscape Bus1/LConn2
  Spatial Contact Force11/LConn1 -- Simscape Bus1/LConn3
  Spatial Contact Force4/LConn1 -- Simscape Bus1/LConn5
  Spatial Contact Force9/LConn1 -- Simscape Bus1/LConn1
  Spatial Contact Force5/LConn1 -- Simscape Bus1/LConn6
  Spatial Contact Force6/LConn1 -- Simscape Bus1/LConn4
  Simscape Bus1/RConn1 -- object/RConn1

== system ship_template/System/object scenario/9objs/contact models/object2object/objectcontact3 ==
  Simscape Bus1 : SimscapeBus  HierarchyStrings=green1;red1;blue2;green2;red2
  Spatial Contact Force{4..6,10..11} (5 alike) : sm_lib/Forces and Torques/Spatial Contact Force  CoefficientOfDynamicFriction=0.3  CoefficientOfStaticFriction=0.5  SenseContactBaseRotation=off  SenseContactBaseTranslation=off  NormalDamping=b  NormalDampingUnits=N/(m/s)  SenseContactFollowerRotation=off  SenseContactFollowerTranslation=off  SenseContactSignal=off  NormalStiffness=k  NormalStiffnessUnits=N/m  FrictionalCriticalVelocity=1e-3  FrictionalCriticalVelocityUnits=m/s  ZeroCrossDetectContactStartAndEnd=off  FrictionType=SmoothStickSlip  SenseFrictionalForceMagnitude=off  SenseNormalForceMagnitude=off  NormalForceType=SmoothSpringDamper  SenseNormalVelocity=off  SenseSeparationDistance=off  SenseTangentialVelocity=off  SenseTangentialVelocityMagnitude=off  NormalTransitionRegionWidth=x  NormalTransitionRegionWidthUnits=m
  object : PMIOPort  Side=Left
  F : PMIOPort  Port=2  Side=Right
  connections:
  Simscape Bus1/LConn5 -- Spatial Contact Force5/LConn1
  Simscape Bus1/LConn1 -- Spatial Contact Force10/LConn1
  Spatial Contact Force5/RConn1 -- Spatial Contact Force10/RConn1 -- Spatial Contact Force11/RConn1 -- Spatial Contact Force6/RConn1 -- Spatial Contact Force4/RConn1 -- F/RConn1
  object/RConn1 -- Simscape Bus1/RConn1
  Simscape Bus1/LConn2 -- Spatial Contact Force11/LConn1
  Simscape Bus1/LConn4 -- Spatial Contact Force4/LConn1
  Simscape Bus1/LConn3 -- Spatial Contact Force6/LConn1

== system ship_template/System/object scenario/9objs/contact models/object2object/objectcontact4 ==
  Simscape Bus1 : SimscapeBus  HierarchyStrings=red1;blue2;green2;red2
  Spatial Contact Force{4..6,11} (4 alike) : sm_lib/Forces and Torques/Spatial Contact Force  CoefficientOfDynamicFriction=0.3  CoefficientOfStaticFriction=0.5  SenseContactBaseRotation=off  SenseContactBaseTranslation=off  NormalDamping=b  NormalDampingUnits=N/(m/s)  SenseContactFollowerRotation=off  SenseContactFollowerTranslation=off  SenseContactSignal=off  NormalStiffness=k  NormalStiffnessUnits=N/m  FrictionalCriticalVelocity=1e-3  FrictionalCriticalVelocityUnits=m/s  ZeroCrossDetectContactStartAndEnd=off  FrictionType=SmoothStickSlip  SenseFrictionalForceMagnitude=off  SenseNormalForceMagnitude=off  NormalForceType=SmoothSpringDamper  SenseNormalVelocity=off  SenseSeparationDistance=off  SenseTangentialVelocity=off  SenseTangentialVelocityMagnitude=off  NormalTransitionRegionWidth=x  NormalTransitionRegionWidthUnits=m
  object : PMIOPort  Side=Left
  F : PMIOPort  Port=2  Side=Right
  connections:
  F/RConn1 -- Spatial Contact Force6/RConn1 -- Spatial Contact Force11/RConn1 -- Spatial Contact Force5/RConn1 -- Spatial Contact Force4/RConn1
  Spatial Contact Force11/LConn1 -- Simscape Bus1/LConn1
  Spatial Contact Force4/LConn1 -- Simscape Bus1/LConn3
  Spatial Contact Force5/LConn1 -- Simscape Bus1/LConn4
  Spatial Contact Force6/LConn1 -- Simscape Bus1/LConn2
  Simscape Bus1/RConn1 -- object/RConn1

== system ship_template/System/object scenario/9objs/contact models/object2object/objectcontact5 ==
  Simscape Bus1 : SimscapeBus  HierarchyStrings=blue2;green2;red2
  Spatial Contact Force4 : sm_lib/Forces and Torques/Spatial Contact Force  CoefficientOfDynamicFriction=0.3  CoefficientOfStaticFriction=0.5  SenseContactBaseRotation=off  SenseContactBaseTranslation=off  NormalDamping=b  NormalDampingUnits=N/(m/s)  SenseContactFollowerRotation=off  SenseContactFollowerTranslation=off  SenseContactSignal=off  NormalStiffness=k  NormalStiffnessUnits=N/m  FrictionalCriticalVelocity=1e-3  FrictionalCriticalVelocityUnits=m/s  ZeroCrossDetectContactStartAndEnd=off  FrictionType=SmoothStickSlip  SenseFrictionalForceMagnitude=off  SenseNormalForceMagnitude=off  NormalForceType=SmoothSpringDamper  SenseNormalVelocity=off  SenseSeparationDistance=off  SenseTangentialVelocity=off  SenseTangentialVelocityMagnitude=off  NormalTransitionRegionWidth=x  NormalTransitionRegionWidthUnits=m
  Spatial Contact Force5 : sm_lib/Forces and Torques/Spatial Contact Force  CoefficientOfDynamicFriction=0.3  CoefficientOfStaticFriction=0.5  SenseContactBaseRotation=off  SenseContactBaseTranslation=off  NormalDamping=b  NormalDampingUnits=N/(m/s)  SenseContactFollowerRotation=off  SenseContactFollowerTranslation=off  SenseContactSignal=off  NormalStiffness=k  NormalStiffnessUnits=N/m  FrictionalCriticalVelocity=1e-3  FrictionalCriticalVelocityUnits=m/s  ZeroCrossDetectContactStartAndEnd=off  FrictionType=SmoothStickSlip  SenseFrictionalForceMagnitude=off  SenseNormalForceMagnitude=off  NormalForceType=SmoothSpringDamper  SenseNormalVelocity=off  SenseSeparationDistance=off  SenseTangentialVelocity=off  SenseTangentialVelocityMagnitude=off  NormalTransitionRegionWidth=x  NormalTransitionRegionWidthUnits=m
  Spatial Contact Force6 : sm_lib/Forces and Torques/Spatial Contact Force  CoefficientOfDynamicFriction=0.3  CoefficientOfStaticFriction=0.5  SenseContactBaseRotation=off  SenseContactBaseTranslation=off  NormalDamping=b  NormalDampingUnits=N/(m/s)  SenseContactFollowerRotation=off  SenseContactFollowerTranslation=off  SenseContactSignal=off  NormalStiffness=k  NormalStiffnessUnits=N/m  FrictionalCriticalVelocity=1e-3  FrictionalCriticalVelocityUnits=m/s  ZeroCrossDetectContactStartAndEnd=off  FrictionType=SmoothStickSlip  SenseFrictionalForceMagnitude=off  SenseNormalForceMagnitude=off  NormalForceType=SmoothSpringDamper  SenseNormalVelocity=off  SenseSeparationDistance=off  SenseTangentialVelocity=off  SenseTangentialVelocityMagnitude=off  NormalTransitionRegionWidth=x  NormalTransitionRegionWidthUnits=m
  object : PMIOPort  Side=Left
  F : PMIOPort  Port=2  Side=Right
  connections:
  Simscape Bus1/RConn1 -- object/RConn1
  Spatial Contact Force6/LConn1 -- Simscape Bus1/LConn1
  Spatial Contact Force5/LConn1 -- Simscape Bus1/LConn3
  Spatial Contact Force4/LConn1 -- Simscape Bus1/LConn2
  Spatial Contact Force6/RConn1 -- Spatial Contact Force5/RConn1 -- F/RConn1 -- Spatial Contact Force4/RConn1

== system ship_template/System/object scenario/9objs/contact models/object2object/objectcontact6 ==
  Simscape Bus1 : SimscapeBus  HierarchyStrings=green2;red2
  Spatial Contact Force4 : sm_lib/Forces and Torques/Spatial Contact Force  CoefficientOfDynamicFriction=0.3  CoefficientOfStaticFriction=0.5  SenseContactBaseRotation=off  SenseContactBaseTranslation=off  NormalDamping=b  NormalDampingUnits=N/(m/s)  SenseContactFollowerRotation=off  SenseContactFollowerTranslation=off  SenseContactSignal=off  NormalStiffness=k  NormalStiffnessUnits=N/m  FrictionalCriticalVelocity=1e-3  FrictionalCriticalVelocityUnits=m/s  ZeroCrossDetectContactStartAndEnd=off  FrictionType=SmoothStickSlip  SenseFrictionalForceMagnitude=off  SenseNormalForceMagnitude=off  NormalForceType=SmoothSpringDamper  SenseNormalVelocity=off  SenseSeparationDistance=off  SenseTangentialVelocity=off  SenseTangentialVelocityMagnitude=off  NormalTransitionRegionWidth=x  NormalTransitionRegionWidthUnits=m
  Spatial Contact Force5 : sm_lib/Forces and Torques/Spatial Contact Force  CoefficientOfDynamicFriction=0.3  CoefficientOfStaticFriction=0.5  SenseContactBaseRotation=off  SenseContactBaseTranslation=off  NormalDamping=b  NormalDampingUnits=N/(m/s)  SenseContactFollowerRotation=off  SenseContactFollowerTranslation=off  SenseContactSignal=off  NormalStiffness=k  NormalStiffnessUnits=N/m  FrictionalCriticalVelocity=1e-3  FrictionalCriticalVelocityUnits=m/s  ZeroCrossDetectContactStartAndEnd=off  FrictionType=SmoothStickSlip  SenseFrictionalForceMagnitude=off  SenseNormalForceMagnitude=off  NormalForceType=SmoothSpringDamper  SenseNormalVelocity=off  SenseSeparationDistance=off  SenseTangentialVelocity=off  SenseTangentialVelocityMagnitude=off  NormalTransitionRegionWidth=x  NormalTransitionRegionWidthUnits=m
  object : PMIOPort  Side=Left
  F : PMIOPort  Port=2  Side=Right
  connections:
  Spatial Contact Force5/RConn1 -- Spatial Contact Force4/RConn1 -- F/RConn1
  Spatial Contact Force4/LConn1 -- Simscape Bus1/LConn1
  Spatial Contact Force5/LConn1 -- Simscape Bus1/LConn2
  Simscape Bus1/RConn1 -- object/RConn1

== system ship_template/System/object scenario/9objs/contact models/object2object/objectcontact7 ==
  Simscape Bus1 : SimscapeBus  HierarchyStrings=red2
  Spatial Contact Force5 : sm_lib/Forces and Torques/Spatial Contact Force  CoefficientOfDynamicFriction=0.3  CoefficientOfStaticFriction=0.5  SenseContactBaseRotation=off  SenseContactBaseTranslation=off  NormalDamping=b  NormalDampingUnits=N/(m/s)  SenseContactFollowerRotation=off  SenseContactFollowerTranslation=off  SenseContactSignal=off  NormalStiffness=k  NormalStiffnessUnits=N/m  FrictionalCriticalVelocity=1e-3  FrictionalCriticalVelocityUnits=m/s  ZeroCrossDetectContactStartAndEnd=off  FrictionType=SmoothStickSlip  SenseFrictionalForceMagnitude=off  SenseNormalForceMagnitude=off  NormalForceType=SmoothSpringDamper  SenseNormalVelocity=off  SenseSeparationDistance=off  SenseTangentialVelocity=off  SenseTangentialVelocityMagnitude=off  NormalTransitionRegionWidth=x  NormalTransitionRegionWidthUnits=m
  object : PMIOPort  Side=Left
  F : PMIOPort  Port=2  Side=Right
  connections:
  Simscape Bus1/RConn1 -- object/RConn1
  Spatial Contact Force5/LConn1 -- Simscape Bus1/LConn1
  Spatial Contact Force5/RConn1 -- F/RConn1
